simulink model "Concurrent_testing"  (R2023b)
settings: Solver=VariableStepAuto  StartTime=0.0  StopTime=600  RelTol=1e-3
undefined symbols (not defined in the file): D, I, N, P
libraries: slpidlib x3
settings Model: Creator=Jack  LastModifiedBy=PC

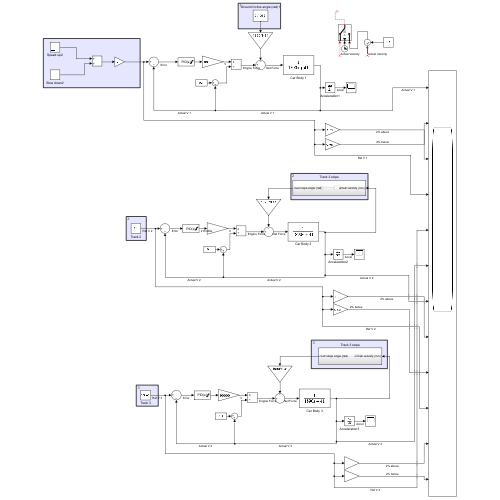
[thumbnail: Simulink's stored preview of the top-level diagram]
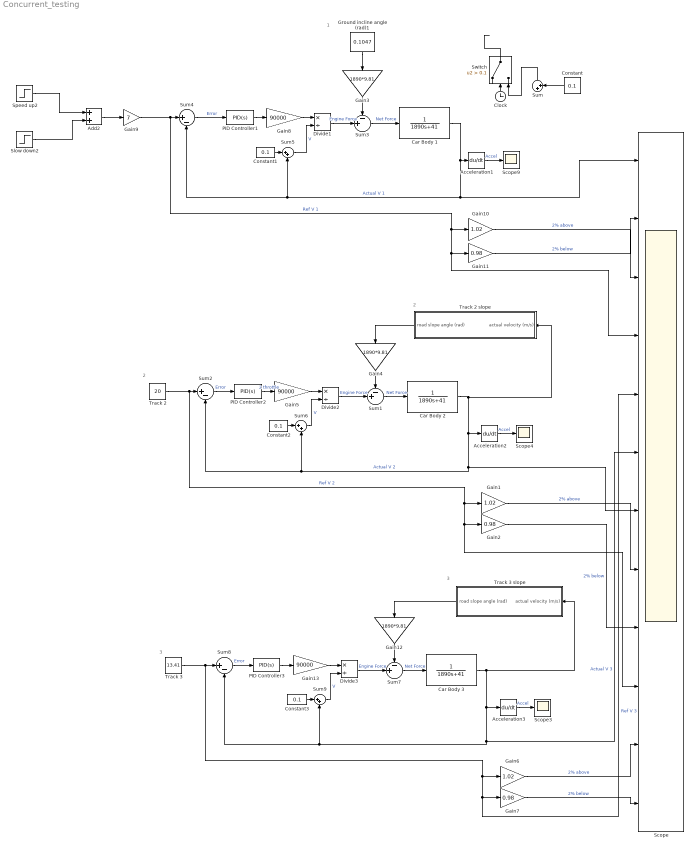
== system Concurrent_testing ==
  note: 1
  note: 2
  note: 2
  note: 3
  note: 3
  Acceleration1 : Derivative
  Acceleration2 : Derivative
  Acceleration3 : Derivative
  Add2 : Sum
  Car Body 1 : TransferFcn  Denominator=[1890 41]
  Car Body 2 : TransferFcn  Denominator=[1890 41]
  Car Body 3 : TransferFcn  Denominator=[1890 41]
  Clock : Clock
  Constant{,1..3} (4 alike) : Constant  Value=0.1
  Divide1 : Product  Inputs=*/
  Divide2 : Product  Inputs=*/
  Divide3 : Product  Inputs=*/
  Gain1 : Gain  Gain=1.02
  Gain10 : Gain  Gain=1.02
  Gain11 : Gain  Gain=0.98
  Gain12 : Gain  Gain=1890*9.81
  Gain13 : Gain  Gain=90000
  Gain2 : Gain  Gain=0.98
  Gain3 : Gain  Gain=1890*9.81
  Gain4 : Gain  Gain=1890*9.81
  Gain5 : Gain  Gain=90000
  Gain6 : Gain  Gain=1.02
  Gain7 : Gain  Gain=0.98
  Gain8 : Gain  Gain=90000
  Gain9 : Gain  Gain=7
  Ground incline angle (rad)1 : Constant  Value=0.1047
  PID Controller1 : slpidlib/PID Controller  Controller=PID  Form=Parallel  TimeDomain=Continuous-time  UseExternalTs=off  SampleTime=-1  IntegratorMethod=Forward Euler  FilterMethod=Forward Euler  ControllerParametersSource=internal  P=P  I=I  UseKiTs=off  D=D  N=N  UseFilter=on  TunerSelectOption=Transfer Function Based (PID Tuner App)  InitialConditionSource=internal  InitialConditionForIntegrator=0  InitialConditionForFilter=0  DifferentiatorICPrevScaledInput=0  ExternalReset=none  TrackingMode=off  Kt=1  LimitOutput=on  SatLimitsSource=internal  UpperSaturationLimit=1  LowerSaturationLimit=-0.3  LinearizeAsGain=on  AntiWindupMode=none  Kb=1  LimitIntegrator=off  UpperIntegratorSaturationLimit=inf  LowerIntegratorSaturationLimit=-inf  POutMin=[]  POutMax=[]  IOutMin=[]  IOutMax=[]  DOutMin=[]  DOutMax=[]  NOutMin=[]  NOutMax=[]  SumOutMin=[]  SumOutMax=[]  SaturationOutMin=[]  SaturationOutMax=[]  PParamMin=[]  PParamMax=[]  IParamMin=[]  IParamMax=[]  DParamMin=[]  DParamMax=[]  NParamMin=[]  NParamMax=[]  KbParamMin=[]  KbParamMax=[]  KtParamMin=[]  KtParamMax=[]  KbOutMin=[]  KbOutMax=[]  KtOutMin=[]  KtOutMax=[]  IntegratorOutMin=[]  IntegratorOutMax=[]  FilterOutMin=[]  FilterOutMax=[]  SumI1OutMin=[]  SumI1OutMax=[]  SumI2OutMin=[]  SumI2OutMax=[]  SumI3OutMin=[]  SumI3OutMax=[]  SumI4OutMin=[]  SumI4OutMax=[]  SumDOutMin=[]  SumDOutMax=[]  DifferentiatorOutMin=[]  DifferentiatorOutMax=[]  FilterDiffOutCoefMin=[]  FilterDiffOutCoefMax=[]  ReciprocalOutMin=[]  ReciprocalOutMax=[]  SumDenOutMin=[]  SumDenOutMax=[]  SumNumOutMin=[]  SumNumOutMax=[]  DivideOutMin=[]  DivideOutMax=[]  UdiffTsProdOutMin=[]  UdiffTsProdOutMax=[]  NTsProdOutMin=[]  NTsProdOutMax=[]  UintegralTsProdOutMin=[]  UintegralTsProdOutMax=[]  UngainTsProdOutMin=[]  UngainTsProdOutMax=[]  ClampingZeroOutDataTypeStr=Inherit: Inherit via back propagation  ClampingZeroOutMin=[]  ClampingZeroOutMax=[]  FilterDenConstantOutDataTypeStr=Inherit: Inherit via back propagation  FilterDenConstantOutMin=[]  FilterDenConstantOutMax=[]  PCopyOutDataTypeStr=Inherit: Inherit via back propagation  PCopyOutMin=[]  PCopyOutMax=[]  NCopyOutDataTypeStr=Inherit: Inherit via back propagation  NCopyOutMin=[]  NCopyOutMax=[]  IntegratorContinuousStateAttributes=''  IntegratorStateMustResolveToSignalObject=off  IntegratorRTWStateStorageClass=Auto  FilterContinuousStateAttributes=''  FilterStateMustResolveToSignalObject=off  FilterRTWStateStorageClass=Auto  ParallelPVariant=InternalParameters  IdealPVariant=Disabled  IVariant=InternalParameters  DVariant=InternalParameters  IntegratorVariant=Continuous  SatVariant=Enabled  AWVariant=Passthrough  PCopyVariant=Disabled  TRVariant=Disabled  FdbkBlocksVariant=Forward  IdealPFdbkVariant=Disabled  SatFdbkVariant=Disabled  DerivativeFilterVariant=ContFilter  NVariant=InternalParameters  NCopyVariant=Disabled  FilterICVariant=InternalICsFilter  IntegratorICVariant=InternalICs  ExternalResetVariant=Disabled  TRSumVariant=Passthrough  SumFdbkVariant=Disabled  SumVariant=Sum_PID  TsampFilterVariant=InternalTs  TsampNgainVariant=Passthrough  TsampIntegralVariant=Disabled_SignalSpec  ExternalSaturationOutDataTypeStr=Inherit: Same as second input
  PID Controller2 : slpidlib/PID Controller  Controller=PID  Form=Parallel  TimeDomain=Continuous-time  UseExternalTs=off  SampleTime=-1  IntegratorMethod=Forward Euler  FilterMethod=Forward Euler  ControllerParametersSource=internal  P=P  I=I  UseKiTs=off  D=D  N=N  UseFilter=on  TunerSelectOption=Transfer Function Based (PID Tuner App)  InitialConditionSource=internal  InitialConditionForIntegrator=0  InitialConditionForFilter=0  DifferentiatorICPrevScaledInput=0  ExternalReset=none  TrackingMode=off  Kt=1  LimitOutput=on  SatLimitsSource=internal  UpperSaturationLimit=1  LowerSaturationLimit=-0.3  LinearizeAsGain=on  AntiWindupMode=none  Kb=1  LimitIntegrator=off  UpperIntegratorSaturationLimit=inf  LowerIntegratorSaturationLimit=-inf  POutMin=[]  POutMax=[]  IOutMin=[]  IOutMax=[]  DOutMin=[]  DOutMax=[]  NOutMin=[]  NOutMax=[]  SumOutMin=[]  SumOutMax=[]  SaturationOutMin=[]  SaturationOutMax=[]  PParamMin=[]  PParamMax=[]  IParamMin=[]  IParamMax=[]  DParamMin=[]  DParamMax=[]  NParamMin=[]  NParamMax=[]  KbParamMin=[]  KbParamMax=[]  KtParamMin=[]  KtParamMax=[]  KbOutMin=[]  KbOutMax=[]  KtOutMin=[]  KtOutMax=[]  IntegratorOutMin=[]  IntegratorOutMax=[]  FilterOutMin=[]  FilterOutMax=[]  SumI1OutMin=[]  SumI1OutMax=[]  SumI2OutMin=[]  SumI2OutMax=[]  SumI3OutMin=[]  SumI3OutMax=[]  SumI4OutMin=[]  SumI4OutMax=[]  SumDOutMin=[]  SumDOutMax=[]  DifferentiatorOutMin=[]  DifferentiatorOutMax=[]  FilterDiffOutCoefMin=[]  FilterDiffOutCoefMax=[]  ReciprocalOutMin=[]  ReciprocalOutMax=[]  SumDenOutMin=[]  SumDenOutMax=[]  SumNumOutMin=[]  SumNumOutMax=[]  DivideOutMin=[]  DivideOutMax=[]  UdiffTsProdOutMin=[]  UdiffTsProdOutMax=[]  NTsProdOutMin=[]  NTsProdOutMax=[]  UintegralTsProdOutMin=[]  UintegralTsProdOutMax=[]  UngainTsProdOutMin=[]  UngainTsProdOutMax=[]  ClampingZeroOutDataTypeStr=Inherit: Inherit via back propagation  ClampingZeroOutMin=[]  ClampingZeroOutMax=[]  FilterDenConstantOutDataTypeStr=Inherit: Inherit via back propagation  FilterDenConstantOutMin=[]  FilterDenConstantOutMax=[]  PCopyOutDataTypeStr=Inherit: Inherit via back propagation  PCopyOutMin=[]  PCopyOutMax=[]  NCopyOutDataTypeStr=Inherit: Inherit via back propagation  NCopyOutMin=[]  NCopyOutMax=[]  IntegratorContinuousStateAttributes=''  IntegratorStateMustResolveToSignalObject=off  IntegratorRTWStateStorageClass=Auto  FilterContinuousStateAttributes=''  FilterStateMustResolveToSignalObject=off  FilterRTWStateStorageClass=Auto  ParallelPVariant=InternalParameters  IdealPVariant=Disabled  IVariant=InternalParameters  DVariant=InternalParameters  IntegratorVariant=Continuous  SatVariant=Enabled  AWVariant=Passthrough  PCopyVariant=Disabled  TRVariant=Disabled  FdbkBlocksVariant=Forward  IdealPFdbkVariant=Disabled  SatFdbkVariant=Disabled  DerivativeFilterVariant=ContFilter  NVariant=InternalParameters  NCopyVariant=Disabled  FilterICVariant=InternalICsFilter  IntegratorICVariant=InternalICs  ExternalResetVariant=Disabled  TRSumVariant=Passthrough  SumFdbkVariant=Disabled  SumVariant=Sum_PID  TsampFilterVariant=InternalTs  TsampNgainVariant=Passthrough  TsampIntegralVariant=Disabled_SignalSpec  ExternalSaturationOutDataTypeStr=Inherit: Same as second input
  PID Controller3 : slpidlib/PID Controller  Controller=PID  Form=Parallel  TimeDomain=Continuous-time  UseExternalTs=off  SampleTime=-1  IntegratorMethod=Forward Euler  FilterMethod=Forward Euler  ControllerParametersSource=internal  P=P  I=I  UseKiTs=off  D=D  N=N  UseFilter=on  TunerSelectOption=Transfer Function Based (PID Tuner App)  InitialConditionSource=internal  InitialConditionForIntegrator=0  InitialConditionForFilter=0  DifferentiatorICPrevScaledInput=0  ExternalReset=none  TrackingMode=off  Kt=1  LimitOutput=on  SatLimitsSource=internal  UpperSaturationLimit=1  LowerSaturationLimit=-0.3  LinearizeAsGain=on  AntiWindupMode=none  Kb=1  LimitIntegrator=off  UpperIntegratorSaturationLimit=inf  LowerIntegratorSaturationLimit=-inf  POutMin=[]  POutMax=[]  IOutMin=[]  IOutMax=[]  DOutMin=[]  DOutMax=[]  NOutMin=[]  NOutMax=[]  SumOutMin=[]  SumOutMax=[]  SaturationOutMin=[]  SaturationOutMax=[]  PParamMin=[]  PParamMax=[]  IParamMin=[]  IParamMax=[]  DParamMin=[]  DParamMax=[]  NParamMin=[]  NParamMax=[]  KbParamMin=[]  KbParamMax=[]  KtParamMin=[]  KtParamMax=[]  KbOutMin=[]  KbOutMax=[]  KtOutMin=[]  KtOutMax=[]  IntegratorOutMin=[]  IntegratorOutMax=[]  FilterOutMin=[]  FilterOutMax=[]  SumI1OutMin=[]  SumI1OutMax=[]  SumI2OutMin=[]  SumI2OutMax=[]  SumI3OutMin=[]  SumI3OutMax=[]  SumI4OutMin=[]  SumI4OutMax=[]  SumDOutMin=[]  SumDOutMax=[]  DifferentiatorOutMin=[]  DifferentiatorOutMax=[]  FilterDiffOutCoefMin=[]  FilterDiffOutCoefMax=[]  ReciprocalOutMin=[]  ReciprocalOutMax=[]  SumDenOutMin=[]  SumDenOutMax=[]  SumNumOutMin=[]  SumNumOutMax=[]  DivideOutMin=[]  DivideOutMax=[]  UdiffTsProdOutMin=[]  UdiffTsProdOutMax=[]  NTsProdOutMin=[]  NTsProdOutMax=[]  UintegralTsProdOutMin=[]  UintegralTsProdOutMax=[]  UngainTsProdOutMin=[]  UngainTsProdOutMax=[]  ClampingZeroOutDataTypeStr=Inherit: Inherit via back propagation  ClampingZeroOutMin=[]  ClampingZeroOutMax=[]  FilterDenConstantOutDataTypeStr=Inherit: Inherit via back propagation  FilterDenConstantOutMin=[]  FilterDenConstantOutMax=[]  PCopyOutDataTypeStr=Inherit: Inherit via back propagation  PCopyOutMin=[]  PCopyOutMax=[]  NCopyOutDataTypeStr=Inherit: Inherit via back propagation  NCopyOutMin=[]  NCopyOutMax=[]  IntegratorContinuousStateAttributes=''  IntegratorStateMustResolveToSignalObject=off  IntegratorRTWStateStorageClass=Auto  FilterContinuousStateAttributes=''  FilterStateMustResolveToSignalObject=off  FilterRTWStateStorageClass=Auto  ParallelPVariant=InternalParameters  IdealPVariant=Disabled  IVariant=InternalParameters  DVariant=InternalParameters  IntegratorVariant=Continuous  SatVariant=Enabled  AWVariant=Passthrough  PCopyVariant=Disabled  TRVariant=Disabled  FdbkBlocksVariant=Forward  IdealPFdbkVariant=Disabled  SatFdbkVariant=Disabled  DerivativeFilterVariant=ContFilter  NVariant=InternalParameters  NCopyVariant=Disabled  FilterICVariant=InternalICsFilter  IntegratorICVariant=InternalICs  ExternalResetVariant=Disabled  TRSumVariant=Passthrough  SumFdbkVariant=Disabled  SumVariant=Sum_PID  TsampFilterVariant=InternalTs  TsampNgainVariant=Passthrough  TsampIntegralVariant=Disabled_SignalSpec  ExternalSaturationOutDataTypeStr=Inherit: Same as second input
  Scope : Scope  NumInputPorts=12
  Scope3 : Scope
  Scope4 : Scope
  Scope9 : Scope
  Slow down2 : Step  Time=300  Before=3  After=2  SampleTime=0
  Speed up2 : Step  Time=50  Before=1  After=3  SampleTime=0
  Sum{,5..6,9} (4 alike) : Sum  Inputs=|++
  Sum1 : Sum  Inputs=-+|
  Sum2 : Sum  Inputs=|+-
  Sum3 : Sum  Inputs=-+|
  Sum4 : Sum  Inputs=|+-
  Sum7 : Sum  Inputs=-+|
  Sum8 : Sum  Inputs=|+-
  Switch : Switch  Criteria=u2 > Threshold  Threshold=0.1  SaturateOnIntegerOverflow=off  InputSameDT=off
  Track 2 : Constant  Value=20
  Track 2 slope : Subsystem
  Track 3 : Constant  Value=13.41
  Track 3 slope : Subsystem
  wires:
  Gain9/1 -> Sum4/1, Scope/4, Gain11/1, Gain10/1  "Ref V 1"
  Sum3/1 -> Car Body 1/1  "Net Force"
  Slow down2/1 -> Add2/2
  Speed up2/1 -> Add2/1
  Gain3/1 -> Sum3/1
  Ground incline angle (rad)1/1 -> Gain3/1
  Gain11/1 -> Scope/2  "2% below"
  Acceleration1/1 -> Scope9/1  "Accel"
  Add2/1 -> Gain9/1
  Constant1/1 -> Sum5/1
  Gain8/1 -> Divide1/1
  Gain10/1 -> Scope/3  "2% above"
  Sum5/1 -> Divide1/2  "V"
  Divide1/1 -> Sum3/2  "Engine Force"
  Car Body 1/1 -> Scope/1, Sum4/2, Sum5/2, Acceleration1/1  "Actual V 1"
  Sum1/1 -> Car Body 2/1  "Net Force"
  Gain4/1 -> Sum1/1
  Gain2/1 -> Scope/9  "2% below"
  Acceleration2/1 -> Scope4/1  "Accel"
  Constant2/1 -> Sum6/1
  Gain5/1 -> Divide2/1
  Gain1/1 -> Scope/8  "2% above"
  Sum6/1 -> Divide2/2  "V"
  Divide2/1 -> Sum1/2  "Engine Force"
  Car Body 2/1 -> Sum2/2, Sum6/2, Scope/7, Acceleration2/1, Track 2 slope/1(actual velocity (m/s))  "Actual V 2"
  Track 2/1 -> Scope/10, Gain2/1, Gain1/1, Sum2/1  "Ref V 2"
  Track 2 slope/1(road slope angle (rad)) -> Gain4/1
  Car Body 3/1 -> Scope/6, Sum8/2, Sum9/2, Acceleration3/1, Track 3 slope/1(actual velocity (m/s))  "Actual V 3"
  Divide3/1 -> Sum7/2  "Engine Force"
  Sum9/1 -> Divide3/2  "V"
  Acceleration3/1 -> Scope3/1  "Accel"
  Gain6/1 -> Scope/11  "2% above"
  Gain12/1 -> Sum7/1
  Gain13/1 -> Divide3/1
  PID Controller3/1 -> Gain13/1
  Constant3/1 -> Sum9/1
  Gain7/1 -> Scope/12  "2% below"
  Sum7/1 -> Car Body 3/1  "Net Force"
  Track 3/1 -> Scope/5, Gain7/1, Gain6/1, Sum8/1  "Ref V 3"
  Track 3 slope/1(road slope angle (rad)) -> Gain12/1
  Sum8/1 -> PID Controller3/1  "Error"
  PID Controller2/1 -> Gain5/1  "2 throttle"
  PID Controller1/1 -> Gain8/1
  Sum2/1 -> PID Controller2/1  "Error"
  Sum4/1 -> PID Controller1/1  "Error"
  Switch/1 -> ?
  Clock/1 -> Switch/2
  Constant/1 -> Sum/2
  Sum/1 -> Switch/3
  ? -> Sum/1  "Actual Velocity"
  ? -> Switch/1  "Actual Velocity"

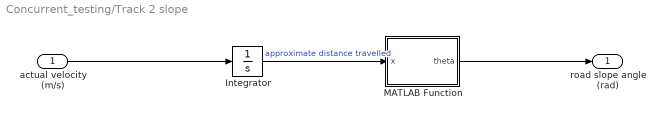
== system Concurrent_testing/Track 2 slope ==
  actual velocity (m/s) : Inport
  Integrator : Integrator
  MATLAB Function : MATLAB Function  TreatAsAtomicUnit=on
  road slope angle (rad) : Outport
  wires:
  MATLAB Function/1(theta) -> road slope angle (rad)/1
  actual velocity (m/s)/1 -> Integrator/1
  Integrator/1 -> MATLAB Function/1(x)  "approximate distance travelled"

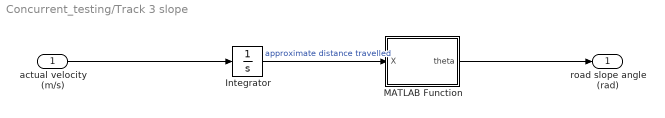
== system Concurrent_testing/Track 3 slope ==
  actual velocity (m/s) : Inport
  Integrator : Integrator
  MATLAB Function : MATLAB Function  TreatAsAtomicUnit=on
  road slope angle (rad) : Outport
  wires:
  MATLAB Function/1(theta) -> road slope angle (rad)/1
  actual velocity (m/s)/1 -> Integrator/1
  Integrator/1 -> MATLAB Function/1(X)  "approximate distance travelled"

== matlab function Concurrent_testing/Track 3 slope/MATLAB Function ==
  data: X input; theta output
function theta = fcn(X)
%CROW_ROAD_(DETAILED) neural network simulation function.
%
% Auto-generated by MATLAB, 13-Feb-2024 14:44:33.
% 
% [Y] = Crow_Road_(detailed)(X,~,~) takes these arguments:
% 
%   X = 1xTS cell, 1 inputs over TS timesteps
%   Each X{1,ts} = 1xQ matrix, input #1 at timestep ts.
% 
% and returns:
%   Y = 1xTS cell of 1 outputs over TS timesteps.
%   Each Y{1,ts} = 1xQ matrix, output #1 at timestep ts.
% 
% where Q is number of samples (or series) and TS is the number of timesteps.

h = 0.01;
Xh = X + h;

XX = X;
XXh = Xh;

% ===== NEURAL NETWORK CONSTANTS =====

% Input 1
Xxoffset = 0;
Xgain = 0.000356346277239324;
Xymin = -1;

% Layer 1
b1 = [-49.290445592277187359;46.599810957157131952;44.566581930010038093;42.50027365885089381;-40.329989883564202557;37.982360207919768413;-36.457279518162216903;33.896652720089257116;-31.570010368637859699;29.063149807387990364;-28.378700570919964008;24.938650481570441286;22.000970304634705599;-20.054073801742063665;18.492568107131560851;-16.350613605858718813;12.389697702441390348;-13.025965079953357062;9.4475638245566386786;7.2010415722369209846;5.5241350240836855079;2.89079098083671715;0.68037339002735253146;1.0838997599094433166;3.0656862746362909533;-6.1990433696652482709;-8.1138715792063749177;-9.8080023157947486823;-12.357415682581500249;-15.052923168286334032;15.62319628067392685;-19.305438375356107628;20.545142476883921034;-23.601579993947030545;24.89349887485881041;-26.590940132895948267;-29.238060133848172484;-31.729278408061123429;-32.979066513614277767;-35.768723184387397396;-38.065922388353328643;40.303630567447356725;-42.523736659229143697;44.592331503960267014;-46.83950547997118008;-48.659946590477289874];
IW1_1 = [48.676077962073648564;-49.160999661643984382;-49.078382728105317767;-49.033488270786889984;48.887258673067144343;-49.047067745236475389;49.77697467108718854;-48.957626160455077979;49.08306153700317509;-48.76988225576507574;51.119476763283529408;-47.78942004219572226;-49.321450006021272827;48.495090520189982897;-49.709563204589642282;49.421365439863315316;-43.675110177514916643;52.566985489046913926;-46.358125697988285197;-47.19922243154532282;-49.634022878091663245;-46.616192478807676025;-49.123515935463601068;48.721694392303930954;49.072273950582825819;-49.093098352183652366;-49.027351452913514152;-48.477212653379680773;-51.744775302813138751;-49.272619526040010385;48.184454373186142107;-48.782060183550335353;48.252853811139573281;-50.367120279288215556;48.788285767898329937;-49.358289829171653196;-48.893632819843048765;-48.516494934888811486;-49.63489323698537703;-48.813345070767830691;-49.055919079822935203;48.90683410895093175;-49.03150185549039719;48.919459009272991068;-49.163030182039022975;-49.267148551038943083];

% Layer 2
b2 = 0.15942743702338207923;
LW2_1 = [0.14457853119386293583 -0.0064465356989518076553 -0.00020166508753487188965 -0.024473095127728550224 0.0085740623474920632519 -0.02545646994293453147 -0.020576290098748867274 -0.032764426612285624252 0.020034191212435707719 0.0064249862653963235593 0.031984163290139075442 -0.00082820947624231977535 -0.016681886350661801616 0.026042403188670959491 0.011895897957470896733 0.038607639328463234929 -0.055363150613066583472 -0.0037614551765473708267 -0.054368667062314260385 -0.054689991670223779552 -0.062388674723919637644 -0.095812072692541230823 -0.039403154958573244349 0.041410213510700316641 0.017806557828306347757 0.0030788927364352181026 -0.0067424008705959589949 -0.076128645849408510538 0.0061982230591948322962 -0.030785508707414935281 0.03249356007364458121 -0.019388634391329755136 0.032787533398445506405 0.026113194748612650331 0.039535105735044831499 -0.019666877092032304664 -0.034913332270165492455 -0.04014780995886310655 -0.018167852518879906015 -0.040055391673606860481 0.01897385071123586231 0.030237916398128630857 0.01134512848458726908 0.031100919974614421593 0.018263777625451727005 0.0016863248588790333282];

% Output 1
Yymin = -1;
Ygain = 0.00739644970414201;
Yxoffset = 66.4;

% ===== SIMULATION ========

% Dimensions
TS = size(X,2); % timesteps
if ~isempty(X)
  Q = size(X(1),2); % samples/series
else
  Q = 0;
end

% Allocate Outputs
Y = zeros(1,TS);
Yh = zeros(1,TS);

% Time loop
for ts=1:TS

    % Input 1
    Xp1 = mapminmax_apply(X(1,ts),Xymin,Xgain,Xxoffset);
    Xhp1 = mapminmax_apply(Xh(1,ts),Xymin,Xgain,Xxoffset);
    
    % Layer 1
    a1 = tansig_apply(repmat(b1,1,Q) + IW1_1*Xp1);
    ah1 = tansig_apply(repmat(b1,1,Q) + IW1_1*Xhp1);
    
    % Layer 2
    a2 = repmat(b2,1,Q) + LW2_1*a1;
    ah2 = repmat(b2,1,Q) + LW2_1*ah1;
    
    % Output 1
    Y(1,ts) = mapminmax_reverse(a2,Yymin,Ygain,Yxoffset);
    Yh(1,ts) = mapminmax_reverse(ah2,Yymin,Ygain,Yxoffset);
end

a = 0; % bumpiness amplitude
b = 2; % bumpiness frequency
Y = Y + a.*sin(XX*b*pi);
Yh = Yh + a.*sin(XXh*b*pi);

theta = atan((Yh-Y)/h); % road inclination [rad]
theta = double(theta);

end

% ===== MODULE FUNCTIONS ========

% Map Minimum and Maximum Input Processing Function
function y = mapminmax_apply(x,ymin,gain,xoffset)
  y = bsxfun(@minus,x,xoffset);
  y = bsxfun(@times,y,gain);
  y = bsxfun(@plus,y,ymin);
end

% Sigmoid Symmetric Transfer Function
function a = tansig_apply(n,~)
  a = 2 ./ (1 + exp(-2*n)) - 1;
end

% Map Minimum and Maximum Output Reverse-Processing Function
function x = mapminmax_reverse(y,ymin,gain,xoffset)
  x = bsxfun(@minus,y,ymin);
  x = bsxfun(@rdivide,x,gain);
  x = bsxfun(@plus,x,xoffset);
end

== matlab function Concurrent_testing/Track 2 slope/MATLAB Function ==
  data: x input; theta output
function theta = fcn(x)

theta = pi/18*exp(0.0001*x)*sin(0.0015*x)*cos(0.001*x)+pi/18;
